simulink model "ysw7_12"  (R2014a)
settings: Solver=ode15s  StartTime=0.0  StopTime=1  RelTol=1e-3
libraries: powerlib x3
settings Model: Creator=Administrator  LastModifiedBy=Administrator

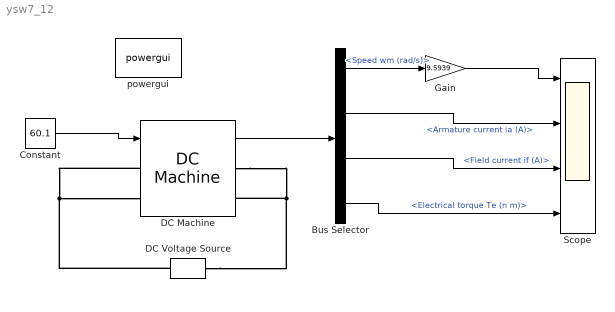
== system ysw7_12 ==
  Bus Selector : BusSelector  OutputSignals=Speed wm (rad/s),Armature current ia (A),Field current if (A),Electrical torque Te (n m)
  Constant : Constant  Value=60.1
  DC Machine : powerlib/Machines/DC Machine  PresetModel=No  MechanicalLoad=Torque TL  FieldType=Wound  ShowDetailedParameters=on  MeasurementBus=off  RLa="[ 0.087  0.0032]"  RLf="[ 181.5  0]"  Laf=0.56  MachineConstant=Torque constant (N.m/A)  Ke=1.8  Kt=1.8  J=0.76  Bm=0  Tf=0  w0=1  Ifinit=1  TsPowergui=0  TsBlock=-1
  DC Voltage Source : powerlib/Electrical Sources/DC Voltage Source  Amplitude=220  Measurements=None
  Gain : Gain  Gain=9.5939
  Scope : Scope  NumInputPorts=4
      settings: YMin=-5~-5~-5~-5  YMax=5~5~5~5
  powergui : powerlib/powergui  Priority=1  SimulationMode=Continuous  SolverType=Tustin  SampleTime=50e-6  frequency=60  SPID=off  DisableSnubberDevices=off  DisableRonSwitches=off  DisableVfSwitches=off  SwTol=0  Interpol=off  DisplayEquations=off  Ts=0  methode=off  frequencyindice=0  Pbase=100e6  ErrMax=1e-4  Iterations=50  UnitsV=kV  UnitsW=MW  FunctionMessages=off  echomessages=off  HookPort=off  EnableUseOfTLC=off  x0status=blocks  RestoreLinks=warning  ResistiveCurrentMeasurement=off  Frange=[0:2:500]  Ylog=off  Xlog=on  ShowGrid=off  save=off  variable=ZData  structure=0  ZoomFFT=off  StartTime=0.0  cycles=1  DisplayStyle=1  fundamental=60  FreqAxis=off  MaxFrequency=1000  frequencyindicesteady=1  RmsSteady=1  display=off
  wires:
  Constant/1 -> DC Machine/1
  Bus Selector/1 -> Gain/1  "<Speed wm (rad/s)>"
  Gain/1 -> Scope/1
  Bus Selector/4 -> Scope/4  "<Electrical torque Te (n m)>"
  DC Machine/1 -> Bus Selector/1
  Bus Selector/3 -> Scope/3  "<Field current if (A)>"
  Bus Selector/2 -> Scope/2  "<Armature current ia (A)>"
  connections:
  DC Voltage Source/RConn1 -- DC Machine/LConn2 -- DC Machine/LConn1
  DC Voltage Source/LConn1 -- DC Machine/RConn2 -- DC Machine/RConn1
